simulink model "Task4_model"  (R2021b)
settings: Solver=VariableStepAuto  StartTime=0.0  StopTime=10.0  RelTol=1e-3
undefined symbols (not defined in the file): K, K_e
settings Model: Creator=witold  LastModifiedBy=witold

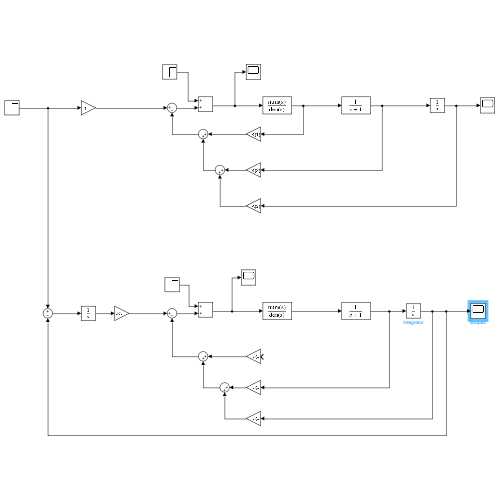
[thumbnail: Simulink's stored preview of the top-level diagram]
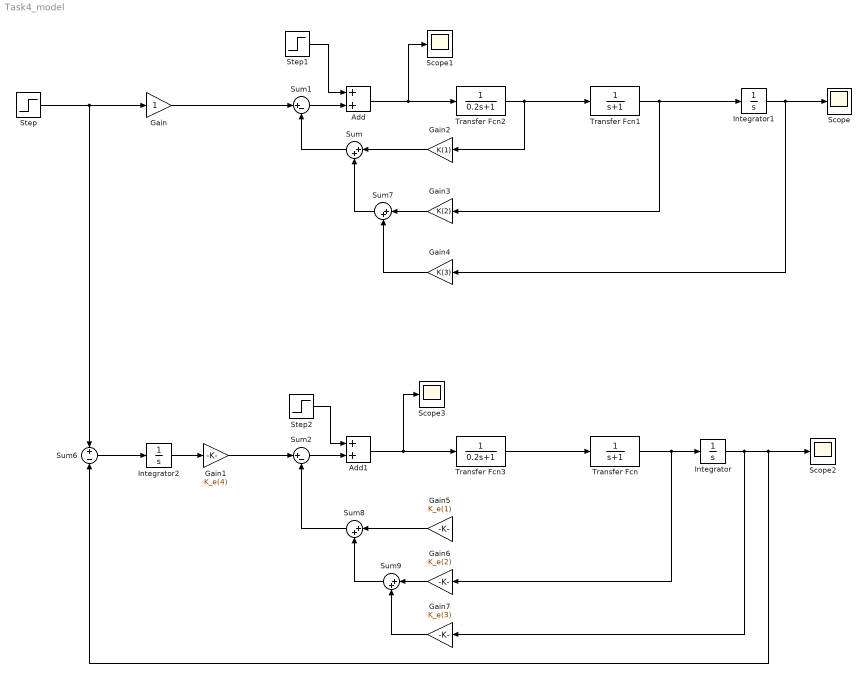
== system Task4_model ==
  Add : Sum
  Add1 : Sum
  Gain : Gain
  Gain1 : Gain  Gain=K_e(4)
  Gain2 : Gain  Gain=K(1)
  Gain3 : Gain  Gain=K(2)
  Gain4 : Gain  Gain=K(3)
  Gain5 : Gain  Gain=K_e(1)
  Gain6 : Gain  Gain=K_e(2)
  Gain7 : Gain  Gain=K_e(3)
  Integrator : Integrator
  Integrator1 : Integrator
  Integrator2 : Integrator
  Scope{,1..3} (4 alike) : Scope
  Step : Step  SampleTime=0
  Step1 : Step  SampleTime=0
  Step2 : Step  SampleTime=0
  Sum{,7..9} (4 alike) : Sum  Inputs=|++
  Sum1 : Sum  Inputs=|+-
  Sum2 : Sum  Inputs=|+-
  Sum6 : Sum  Inputs=+-
  Transfer Fcn : TransferFcn  Denominator=[1 1]
  Transfer Fcn1 : TransferFcn  Denominator=[1 1]
  Transfer Fcn2 : TransferFcn  Denominator=[0.2 1]
  Transfer Fcn3 : TransferFcn  Denominator=[0.2 1]
  wires:
  Step/1 -> Sum6/1, Gain/1
  Gain/1 -> Sum1/1
  Sum/1 -> Sum1/2
  Sum7/1 -> Sum/2
  Gain2/1 -> Sum/1
  Gain3/1 -> Sum7/1
  Gain4/1 -> Sum7/2
  Sum1/1 -> Add/2
  Step1/1 -> Add/1
  Add/1 -> Scope1/1, Transfer Fcn2/1
  Transfer Fcn2/1 -> Transfer Fcn1/1, Gain2/1
  Transfer Fcn1/1 -> Integrator1/1, Gain3/1
  Integrator1/1 -> Scope/1, Gain4/1
  Integrator2/1 -> Gain1/1
  Sum6/1 -> Integrator2/1
  Gain1/1 -> Sum2/1
  Gain5/1 -> Sum8/1
  Gain6/1 -> Sum9/1
  Sum9/1 -> Sum8/2
  Gain7/1 -> Sum9/2
  Sum8/1 -> Sum2/2
  Sum2/1 -> Add1/2
  Step2/1 -> Add1/1
  Add1/1 -> Scope3/1, Transfer Fcn3/1
  Transfer Fcn3/1 -> Transfer Fcn/1
  Transfer Fcn/1 -> Gain6/1, Integrator/1
  Integrator/1 -> Scope2/1, Sum6/2, Gain7/1
